simulink model "demo_Plant_EnergyArb_24_100h"  (R2025b)
settings: Solver=ode15s  StartTime=0.0  StopTime=172800  MaxStep=60  RelTol=1e-3
undefined symbols (not defined in the file): ironair_demo_schedule
libraries: lib_IronAir x5
settings Model: Creator=admin  LastModifiedBy=admin

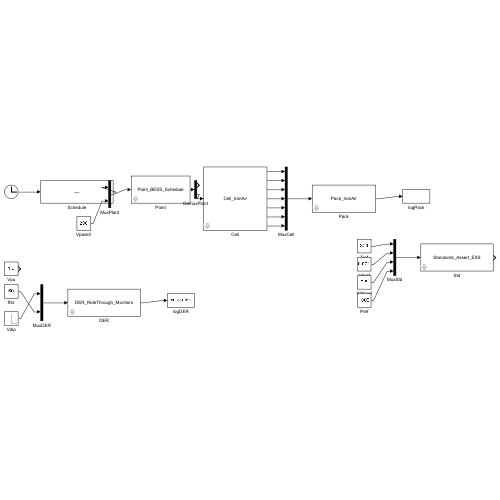
[thumbnail: Simulink's stored preview of the top-level diagram]
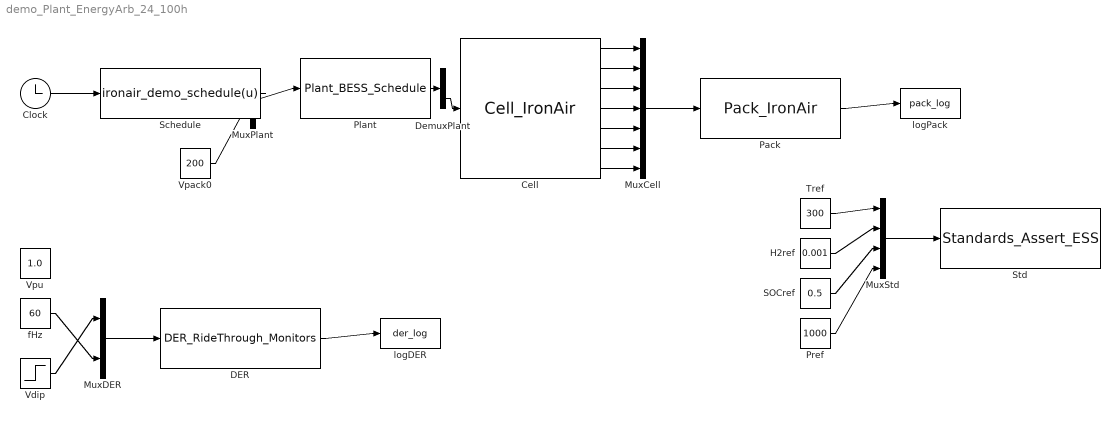
== system demo_Plant_EnergyArb_24_100h ==
  Cell : lib_IronAir/Cell_IronAir
  Clock : Clock
  DER : lib_IronAir/DER_RideThrough_Monitors
  DemuxPlant : Demux  Outputs=2
  H2ref : Constant  Value=0.001
  MuxCell : Mux  Inputs=7
  MuxDER : Mux  Inputs=2
  MuxPlant : Mux  Inputs=2
  MuxStd : Mux
  Pack : lib_IronAir/Pack_IronAir
  Plant : lib_IronAir/Plant_BESS_Schedule
  Pref : Constant  Value=1000
  SOCref : Constant  Value=0.5
  Schedule : MATLABFcn  MATLABFcn=ironair_demo_schedule(u)  OutputDimensions=1
  Std : lib_IronAir/Standards_Assert_ESS
  Tref : Constant  Value=300
  Vdip : Step  Time=3600*6  Before=1.0  After=0.85  SampleTime=0
  Vpack0 : Constant  Value=200
  Vpu : Constant  Value=1.0
  fHz : Constant  Value=60
  logDER : ToWorkspace  VariableName=der_log  SaveFormat=Timeseries  SampleTime=-1
  logPack : ToWorkspace  VariableName=pack_log  SaveFormat=Timeseries  SampleTime=-1
  wires:
  Clock/1 -> Schedule/1
  Schedule/1 -> MuxPlant/1
  Vpack0/1 -> MuxPlant/2
  MuxPlant/1 -> Plant/1
  Plant/1 -> DemuxPlant/1
  DemuxPlant/2 -> Cell/1
  Cell/1 -> MuxCell/1
  Cell/2 -> MuxCell/2
  Cell/3 -> MuxCell/3
  Cell/4 -> MuxCell/4
  Cell/5 -> MuxCell/5
  Cell/6 -> MuxCell/6
  Cell/7 -> MuxCell/7
  MuxCell/1 -> Pack/1
  Pack/1 -> logPack/1
  Vdip/1 -> MuxDER/1
  fHz/1 -> MuxDER/2
  MuxDER/1 -> DER/1
  DER/1 -> logDER/1
  Tref/1 -> MuxStd/1
  H2ref/1 -> MuxStd/2
  SOCref/1 -> MuxStd/3
  Pref/1 -> MuxStd/4
  MuxStd/1 -> Std/1
